simulink model "Thruster"  (R2019b)
settings: Solver=VariableStepAuto  StartTime=0.0  StopTime=10.0  RelTol=1e-3
undefined symbols (not defined in the file): w0_neg, w0_pos, w1_neg, w1_pos, w2_neg, w2_pos
settings Model: Creator=lbend  LastModifiedBy=lbend
settings DebuggingCC: UnconnectedInputMsg=none  UnconnectedOutputMsg=none  UnconnectedLineMsg=none  SFMachineParentedDataDiag=error
settings ModelReferenceCC: EnableRefExpFcnMdlSchedulingChecks=off
settings RTWCC: Description=Generic Real-Time Target

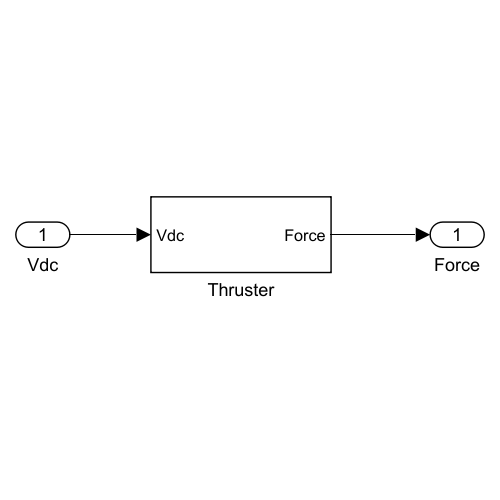
[thumbnail: Simulink's stored preview of the top-level diagram]
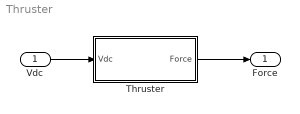
== system Thruster ==
  Vdc : Inport
  Thruster : Subsystem
  Force : Outport
  wires:
  Vdc/1 -> Thruster/1(Vdc)
  Thruster/1(Force) -> Force/1

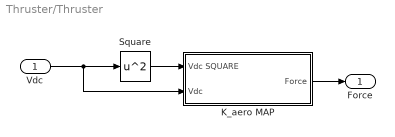
== system Thruster/Thruster ==
  Vdc : Inport
  K_aero MAP : Subsystem
  Square : Math  Operator=square  SaturateOnIntegerOverflow=on
  Force : Outport
  wires:
  Vdc/1 -> K_aero MAP/2(Vdc), Square/1
  Square/1 -> K_aero MAP/1(Vdc SQUARE)
  K_aero MAP/1(Force) -> Force/1

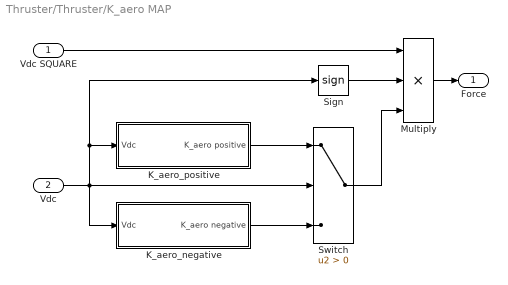
== system Thruster/Thruster/K_aero MAP ==
  Vdc SQUARE : Inport
  Vdc : Inport  Port=2
  K_aero_negative : Subsystem
  K_aero_positive : Subsystem
  "Multiply " : Product  Inputs=***
  Sign : Signum
  Switch : Switch  Criteria=u2 > Threshold
  Force : Outport
  wires:
  Vdc SQUARE/1 -> "Multiply "/1
  "Multiply "/1 -> Force/1
  Vdc/1 -> K_aero_negative/1(Vdc), Switch/2, Sign/1, K_aero_positive/1(Vdc)
  K_aero_positive/1(K_aero positive) -> Switch/1
  K_aero_negative/1(K_aero negative) -> Switch/3
  Switch/1 -> "Multiply "/3
  Sign/1 -> "Multiply "/2

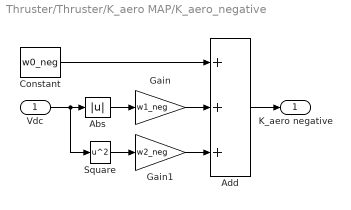
== system Thruster/Thruster/K_aero MAP/K_aero_negative ==
  Vdc : Inport
  Abs : Abs
  Add : Sum  Inputs=+++
  Constant : Constant  Value=w0_neg
  Gain : Gain  Gain=w1_neg
  Gain1 : Gain  Gain=w2_neg
  Square : Math  Operator=square  SaturateOnIntegerOverflow=on
  K_aero negative : Outport
  wires:
  Gain1/1 -> Add/3
  Add/1 -> K_aero negative/1
  Constant/1 -> Add/1
  Gain/1 -> Add/2
  Square/1 -> Gain1/1
  Abs/1 -> Gain/1
  Vdc/1 -> Square/1, Abs/1

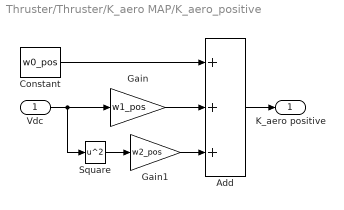
== system Thruster/Thruster/K_aero MAP/K_aero_positive ==
  Vdc : Inport
  Add : Sum  Inputs=+++
  Constant : Constant  Value=w0_pos
  Gain : Gain  Gain=w1_pos
  Gain1 : Gain  Gain=w2_pos
  Square : Math  Operator=square  SaturateOnIntegerOverflow=on
  K_aero positive : Outport
  wires:
  Constant/1 -> Add/1
  Vdc/1 -> Square/1, Gain/1
  Add/1 -> K_aero positive/1
  Gain/1 -> Add/2
  Square/1 -> Gain1/1
  Gain1/1 -> Add/3
